simulink model "wbs_sim"  (R2025a)
settings: Solver=FixedStepAuto  StartTime=0.0  StopTime=20  FixedStep=0.001  RelTol=1e-3
undefined symbols (not defined in the file): dyaw, L_l, L_r, phi_1l, phi_1r, phi_4l, phi_4r, roll, theta_l, theta_r, x, X, Y, yaw, Z
libraries: sm_lib x86, nesl_utility x28, slpidlib x6
(part 4 of 4)

== matlab function wbs_sim/controller/leg controller/right leg feedforward ==
  data: theta input; feedforward output
function feedforward = FFdf(theta)
%FFdf
%    FEEDFORWARD = FFdf(THETA)

%    This function was generated by the Symbolic Math Toolbox version 25.1.
%    2025-12-06 00:25:32

feedforward = (6.37e+2./1.0e+1)./cos(theta);
end
